simulink model "ACA"  (R2018a)
settings: Solver=FixedStepAuto  StartTime=0.0  StopTime=1000  FixedStep=dt  RelTol=1e-3
InitFcn:
  | ACA_init
values from neighbouring files (symbols this model uses):
  G = [eye(5);-eye(5)]    [dir_alloc_sim.m]
  INDX = IN_MAT(k+3,1:m)'    [DAwrap.m]    (also in LPwrap.m = IN_MAT(end,1:m)'; LPwrap_1.m; TESTac.m = zeros(1,NumU); getUperp.m = IN_MAT(end,:)>0.5)
  LPmethod = 0    [LPwrap.m]    (also in LPwrap_1.m; TESTac.m = 10; test.m = 13)
  NumU = 16    [TESTac.m]    (also in test.m)
  uMax = uMax-ue    [DPnewprio_LPCA.m]    (also in DPscaledprio_LPCA.m; LPwrap.m = umax_act; LPwrap_1.m = umax_act; LPwraparm.m = IN_MAT(5,1:4)')
  uMin = uMin-ue    [DPnewprio_LPCA.m]    (also in DPscaledprio_LPCA.m; LPwrap.m = umin_act; LPwrap_1.m = umin_act; LPwraparm.m = IN_MAT(4,1:4)')
undefined symbols (not defined in the file or in its folder): CAmethod, CB, CGIwrap, d2r, DAwrap, DiscIntNeverNeededParam, dt, LPwrap, M_des, PD_max, PD_min, r2d, u0new, u_max, u_min, UD_max, UD_min, Urlim, UseRL, VD_max, VD_min, VJAwrap, WD_max, WD_min, Wp_aca
libraries: simulink x6
settings Model: Creator=Meng Chaoheng  LastModifiedBy=Meng Chaoheng
settings ModelReferenceCC: ModelReferenceNumInstancesAllowed=Single

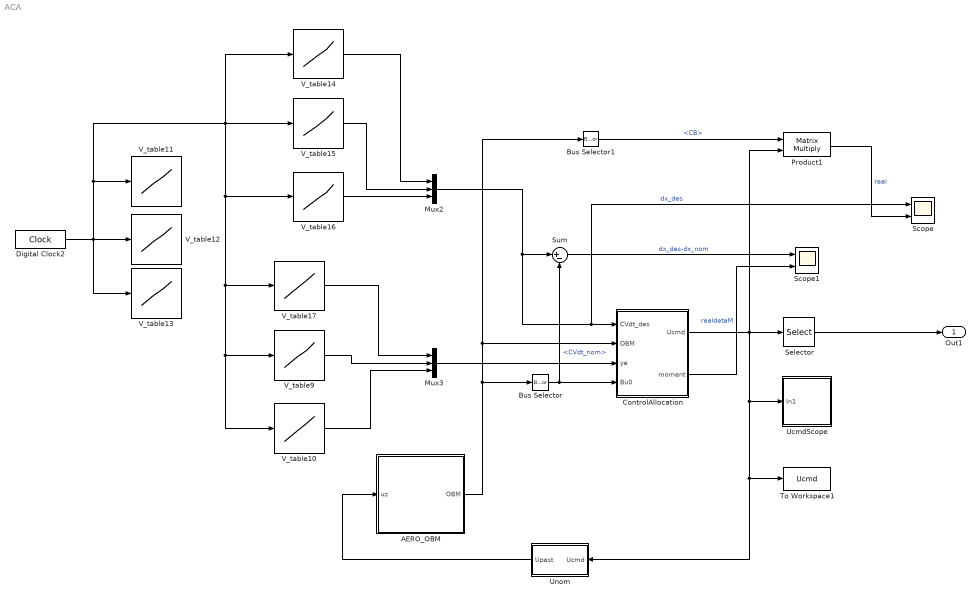
== system ACA ==
  AERO_OBM : Subsystem
  Bus Selector : BusSelector  OutputSignals=CVdt_nom
  Bus Selector1 : BusSelector  OutputSignals=CB
  ControlAllocation : Subsystem
  Digital Clock2 : DigitalClock  SampleTime=dt
  Mux2 : Mux  Inputs=3
  Mux3 : Mux  Inputs=3
  Product1 : Product  Inputs=**  Multiplication=Matrix(*)  RndMeth=Zero
  Scope : Scope  NumInputPorts=2
  Scope1 : Scope  NumInputPorts=2
  Selector : Selector  InputPortWidth=16  IndexOptions=Index vector (dialog)  Indices=[1:4]  OutputSizes=1
  Sum : Sum  Inputs=|+-
  To Workspace1 : ToWorkspace  VariableName=Ucmd  SampleTime=-1
  UcmdScope : Subsystem
  Unom : Subsystem
  V_table10 : Lookup  InputValues=t  Table=ones(length(t),1)*0.0  LookUpMeth=Interpolation-Use End Values
  V_table11 : Lookup  InputValues=t  Table=M_des(:,1)  LookUpMeth=Interpolation-Use End Values
  V_table12 : Lookup  InputValues=t  Table=M_des(:,2)  LookUpMeth=Interpolation-Use End Values
  V_table13 : Lookup  InputValues=t  Table=M_des(:,3)  LookUpMeth=Interpolation-Use End Values
  V_table14 : Lookup  InputValues=t  Table=0.2*sin(0.01*pi*t)  LookUpMeth=Interpolation-Use End Values
  V_table15 : Lookup  InputValues=t  Table=0.2*cos(0.01*pi*t)  LookUpMeth=Interpolation-Use End Values
  V_table16 : Lookup  InputValues=t  Table=0.0*cos(0.02*pi*t)  LookUpMeth=Interpolation-Use End Values
  V_table17 : Lookup  InputValues=t  Table=ones(length(t),1)*0  LookUpMeth=Interpolation-Use End Values
  V_table9 : Lookup  InputValues=t  Table=ones(length(t),1)*0  LookUpMeth=Interpolation-Use End Values
  Out1 : Outport
  wires:
  Unom/1(Upast) -> AERO_OBM/1(uz)
  ControlAllocation/2(moment) -> Scope1/2  "realdetaM"
  Bus Selector/1 -> ControlAllocation/4(Bu0), Sum/2  "<CVdt_nom>"
  AERO_OBM/1(OBM) -> ControlAllocation/2(OBM), Bus Selector1/1, Bus Selector/1
  Bus Selector1/1 -> Product1/1  "<CB>"
  Product1/1 -> Scope/2  "real"
  ControlAllocation/1(Ucmd) -> Product1/2, Selector/1, To Workspace1/1, Unom/1(Ucmd), UcmdScope/1(In1)
  Selector/1 -> Out1/1
  Sum/1 -> Scope1/1  "dx_des-dx_nom"
  Mux3/1 -> ControlAllocation/3(ye)
  Mux2/1 -> ControlAllocation/1(CVdt_des), Scope/1, Sum/1  "dx_des"
  V_table9/1 -> Mux3/2
  V_table17/1 -> Mux3/1
  Digital Clock2/1 -> V_table14/1, V_table15/1, V_table16/1, V_table10/1, V_table9/1, V_table17/1, V_table11/1, V_table13/1, V_table12/1
  V_table14/1 -> Mux2/1
  V_table10/1 -> Mux3/3
  V_table15/1 -> Mux2/2
  V_table16/1 -> Mux2/3

== system ACA/AERO_OBM ==
  uz : Inport
  AeroLimits : Subsystem
  Bus Creator1 : BusCreator  Inputs=5
  Bus Selector : BusSelector  OutputSignals=Unom
  LinearOBM : Subsystem
  OBM : Outport
  wires:
  AeroLimits/1(Umin) -> Bus Creator1/4
  AeroLimits/2(Umax) -> Bus Creator1/5
  Bus Creator1/1 -> OBM/1
  uz/1 -> Bus Selector/1
  Bus Selector/1 -> LinearOBM/1(Unom), Bus Creator1/3  "<Unom>"
  LinearOBM/1(CVdt_nom) -> Bus Creator1/1
  LinearOBM/2(CB) -> Bus Creator1/2

== system ACA/ControlAllocation ==
  CVdt_des : Inport
  OBM : Inport  Port=2
  ye : Inport  Port=3
  Bu0 : Inport  Port=4
  Bus Selector : BusSelector  OutputSignals=CB
  GetU : Subsystem
  PostProcess : Subsystem
  PreProcess : Subsystem
  Product1 : Product  Inputs=**  Multiplication=Matrix(*)  RndMeth=Zero
  Ucmd : Outport
  moment : Outport  Port=2
  wires:
  PreProcess/1(PrePro) -> GetU/1(PrePro), PostProcess/2(PrePro)
  GetU/1(u) -> PostProcess/1(u), Product1/2
  CVdt_des/1 -> PreProcess/1(CVdt_des)  "CVdt_des"
  OBM/1 -> PreProcess/2(OBM), Bus Selector/1
  PostProcess/1(Ucmd) -> Ucmd/1
  Bus Selector/1 -> Product1/1  "<CB>"
  Product1/1 -> moment/1
  ye/1 -> GetU/2(ye)
  Bu0/1 -> GetU/3(Bu0)

== system ACA/UcmdScope ==
  In1 : Inport
  Demux : Demux  Outputs=7
  Selector : Selector  InputPortWidth=16  IndexOptions=Index vector (dialog)  Indices=[1:7]  OutputSizes=1
  Ucmd_deg : Scope  NumInputPorts=7
  scale1 : Gain  Gain=r2d
  wires:
  Selector/1 -> scale1/1
  scale1/1 -> Demux/1
  In1/1 -> Selector/1
  Demux/2 -> Ucmd_deg/2  "LC_deg"
  Demux/1 -> Ucmd_deg/1  "RC_deg"
  Demux/5 -> Ucmd_deg/5  "LIE_deg"
  Demux/7 -> Ucmd_deg/7  "RUD_deg"
  Demux/6 -> Ucmd_deg/6  "LOE_deg"
  Demux/3 -> Ucmd_deg/3  "ROE_deg"
  Demux/4 -> Ucmd_deg/4  "RIE_deg"

== system ACA/Unom ==
  Ucmd : Inport
  Bus Creator : BusCreator  Inputs=2
  Discrete-Time Integrator : DiscreteIntegrator  IntegratorMethod=Integration: Trapezoidal  InitialCondition=u0new  SampleTime=dt  ICPrevOutput=DiscIntNeverNeededParam  ICPrevScaledInput=DiscIntNeverNeededParam
  Get_Unom : Subsystem
  Sum2 : Sum  Inputs=|+-
  Unit Delay1 : UnitDelay  InitialCondition=u0new  SampleTime=dt
  Unit Delay2 : UnitDelay  InitialCondition=u0new  SampleTime=dt
  scale1 : Gain
  scale2 : Gain  Gain=20
  Upast : Outport
  wires:
  Discrete-Time Integrator/1 -> scale1/1, Unit Delay2/1
  Unit Delay1/1 -> Sum2/1, Get_Unom/2(Uz)
  Sum2/1 -> scale2/1
  Unit Delay2/1 -> Sum2/2
  scale2/1 -> Discrete-Time Integrator/1
  Ucmd/1 -> Unit Delay1/1
  scale1/1 -> Get_Unom/1(Uact), Bus Creator/1  "Uact"
  Get_Unom/1(Unom) -> Bus Creator/2
  Bus Creator/1 -> Upast/1

== system ACA/AERO_OBM/AeroLimits ==
  get_uMax : Constant  Value=uMax
  get_uMin : Constant  Value=uMin
  Umin : Outport
  Umax : Outport  Port=2
  wires:
  get_uMin/1 -> Umin/1  "Umin"
  get_uMax/1 -> Umax/1  "Umax"

== system ACA/AERO_OBM/LinearOBM ==
  Unom : Inport
  CB_const : Constant  Value=CB
  Product1 : Product  Inputs=**  Multiplication=Matrix(*)  RndMeth=Zero
  Signal Specification1 : SignalSpecification  Dimensions=[NumU 1]
  CVdt_nom : Outport
  CB : Outport  Port=2
  wires:
  CB_const/1 -> Product1/1, CB/1  "CB"
  Unom/1 -> Signal Specification1/1
  Product1/1 -> CVdt_nom/1  "CVdt_nom"
  Signal Specification1/1 -> Product1/2

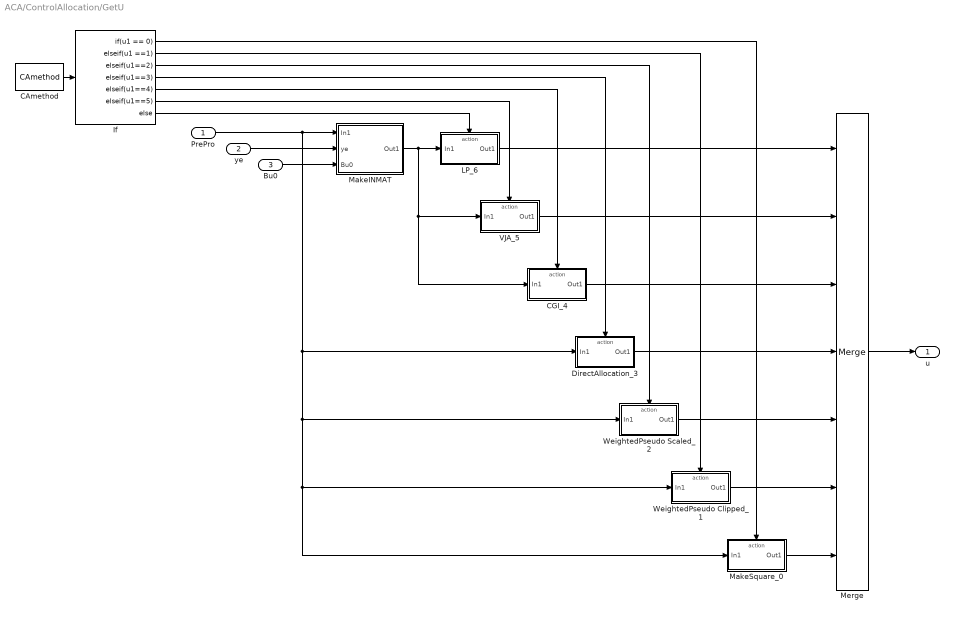
== system ACA/ControlAllocation/GetU ==
  PrePro : Inport
  ye : Inport  Port=2
  Bu0 : Inport  Port=3
  CAmethod : Constant  Value=CAmethod  OutDataTypeStr=int8
  CGI_4 : Subsystem  TreatAsAtomicUnit=on
  DirectAllocation_3 : Subsystem  TreatAsAtomicUnit=on
  If : If  IfExpression=u1 == 0  ElseIfExpressions=u1 ==1, u1==2, u1==3, u1==4, u1==5
  LP_6 : Subsystem  TreatAsAtomicUnit=on
  MakeINMAT : Subsystem
  MakeSquare_0 : Subsystem  TreatAsAtomicUnit=on
  Merge : Merge  Inputs=7
  VJA_5 : Subsystem  TreatAsAtomicUnit=on
  WeightedPseudo Clipped_1 : Subsystem  TreatAsAtomicUnit=on
  WeightedPseudo Scaled_2 : Subsystem  TreatAsAtomicUnit=on
  u : Outport
  wires:
  CAmethod/1 -> If/1
  If/1 -> MakeSquare_0/Action
  If/2 -> WeightedPseudo Clipped_1/Action
  If/3 -> WeightedPseudo Scaled_2/Action
  If/4 -> DirectAllocation_3/Action
  VJA_5/1(Out1) -> Merge/2
  MakeSquare_0/1(Out1) -> Merge/7
  WeightedPseudo Clipped_1/1(Out1) -> Merge/6
  WeightedPseudo Scaled_2/1(Out1) -> Merge/5
  DirectAllocation_3/1(Out1) -> Merge/4
  If/5 -> CGI_4/Action
  CGI_4/1(Out1) -> Merge/3
  If/6 -> VJA_5/Action
  Merge/1 -> u/1
  If/7 -> LP_6/Action
  LP_6/1(Out1) -> Merge/1
  PrePro/1 -> DirectAllocation_3/1(In1), WeightedPseudo Scaled_2/1(In1), WeightedPseudo Clipped_1/1(In1), MakeSquare_0/1(In1), MakeINMAT/1(In1)
  MakeINMAT/1(Out1) -> LP_6/1(In1), VJA_5/1(In1), CGI_4/1(In1)
  ye/1 -> MakeINMAT/2(ye)
  Bu0/1 -> MakeINMAT/3(Bu0)

== system ACA/ControlAllocation/PostProcess ==
  u : Inport
  PrePro : Inport  Port=2
  Bus Selector1 : BusSelector  OutputSignals=Unom
  DriveToPreferred : Subsystem
  Sum2 : Sum  Inputs=|++
  Sum3 : Sum  Inputs=|++
  limits : Subsystem
  Ucmd : Outport
  wires:
  Sum2/1 -> Sum3/1
  u/1 -> DriveToPreferred/2(u), Sum2/1  "u_cmd-u_nom"
  PrePro/1 -> Bus Selector1/1, DriveToPreferred/1(PrePro)
  limits/1(Ucmd) -> Ucmd/1
  Bus Selector1/1 -> Sum2/2  "<Unom>"
  Sum3/1 -> limits/1(In1)
  DriveToPreferred/1(Out2) -> ?

== system ACA/ControlAllocation/PreProcess ==
  CVdt_des : Inport
  OBM : Inport  Port=2
  Bus Creator : BusCreator  Inputs=6
  Bus Selector : BusSelector  OutputSignals=CB
  Bus Selector2 : BusSelector  OutputSignals=Unom
  Constant : Constant  Value=INDX
  GetLimits : Subsystem
  PrePro : Outport
  wires:
  CVdt_des/1 -> Bus Creator/1
  OBM/1 -> Bus Selector/1, Bus Selector2/1, GetLimits/1(OBM)
  Bus Selector/1 -> Bus Creator/2  "<CB>"
  Bus Creator/1 -> PrePro/1
  Bus Selector2/1 -> Bus Creator/3  "<Unom>"
  GetLimits/1(Umin) -> Bus Creator/4
  GetLimits/2(Umax) -> Bus Creator/5
  Constant/1 -> Bus Creator/6  "INDX"

== system ACA/Unom/Get_Unom ==
  note: 2.最优化方法，u_nom是分配起点，
      | 对于典型的QP法，如WLS，SLS等，不要求变量过零，u_nom任意，约束任意，通常无恢复问题（最小范数已经在代价函数中）。
      | 对于LP法，最优化方程的约束只有变量，类似典型QP，约束有方向保持的DP问题：
      | 1）如果u_nom是变化的，即逐帧运行，LP方法有回零恢复问题需要恢复模块（代价函数只优化一帧时）。速度约束可选。
      | 2）如果u_nom是固定点，即全局问题，DP不能加速度约束（不过零）。不需要re可回零，但re可让某些实现的输出曲线更圆滑。
  note: 1.几何法，不考虑约束，和u_nom无关。
  Uact : Inport
  Uz : Inport  Port=2
  Constant3 : Constant  OutDataTypeStr=int8
  Multiport Switch : MultiPortSwitch  Inputs=4
  Utrim : Constant  Value=u0new
  Uzero : Constant  Value=zeros(16,1)
  Unom : Outport
  wires:
  Multiport Switch/1 -> Unom/1  "Unom"
  Constant3/1 -> Multiport Switch/1
  Uzero/1 -> Multiport Switch/2  "Set the nominal values to zero"
  Utrim/1 -> Multiport Switch/3  "Trim the aircraft and use the trimmed values"
  Uz/1 -> Multiport Switch/4  "last computed command"
  Uact/1 -> Multiport Switch/5  "Use the last computed command sent through an estimated effector transfer function"

== system ACA/ControlAllocation/GetU/CGI_4 ==
  In1 : Inport
  Action Port : ActionPort  ActionType=elseif
  MATLAB Fcn : MATLABFcn  MATLABFcn=CGIwrap(u)
  Out1 : Outport
  wires:
  MATLAB Fcn/1 -> Out1/1
  In1/1 -> MATLAB Fcn/1

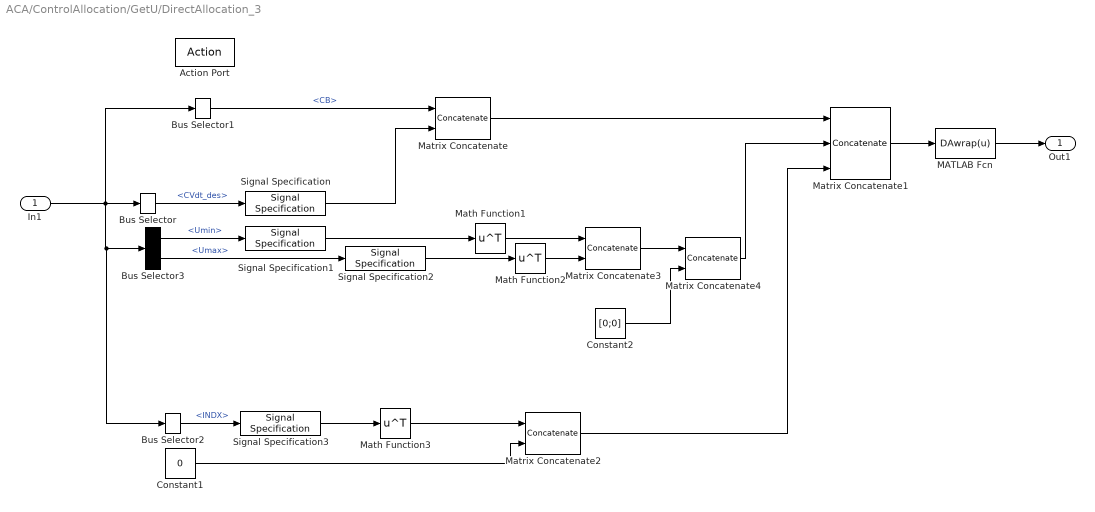
== system ACA/ControlAllocation/GetU/DirectAllocation_3 ==
  In1 : Inport
  Action Port : ActionPort  ActionType=elseif
  Bus Selector : BusSelector  OutputSignals=CVdt_des
  Bus Selector1 : BusSelector  OutputSignals=CB
  Bus Selector2 : BusSelector  OutputSignals=INDX
  Bus Selector3 : BusSelector  OutputSignals=Umin,Umax
  Constant1 : Constant  Value=0
  Constant2 : Constant  Value=[0;0]
  MATLAB Fcn : MATLABFcn  MATLABFcn=DAwrap(u)
  Math Function1 : Math  Operator=transpose  SaturateOnIntegerOverflow=on
  Math Function2 : Math  Operator=transpose  SaturateOnIntegerOverflow=on
  Math Function3 : Math  Operator=transpose  SaturateOnIntegerOverflow=on
  Matrix Concatenate : Concatenate  Mode=Multidimensional array  ConcatenateDimension=2
  Matrix Concatenate1 : Concatenate  NumInputs=3  Mode=Multidimensional array
  Matrix Concatenate2 : Concatenate  Mode=Multidimensional array  ConcatenateDimension=2
  Matrix Concatenate3 : Concatenate  Mode=Multidimensional array
  Matrix Concatenate4 : Concatenate  Mode=Multidimensional array  ConcatenateDimension=2
  Signal Specification : SignalSpecification  Dimensions=[3 1]
  Signal Specification1 : SignalSpecification  Dimensions=[NumU 1]
  Signal Specification2 : SignalSpecification  Dimensions=[NumU 1]
  Signal Specification3 : SignalSpecification  Dimensions=[NumU 1]
  Out1 : Outport
  wires:
  MATLAB Fcn/1 -> Out1/1
  In1/1 -> Bus Selector/1, Bus Selector1/1, Bus Selector2/1, Bus Selector3/1
  Bus Selector/1 -> Signal Specification/1  "<CVdt_des>"
  Bus Selector1/1 -> Matrix Concatenate/1  "<CB>"
  Matrix Concatenate/1 -> Matrix Concatenate1/1
  Matrix Concatenate4/1 -> Matrix Concatenate1/2
  Signal Specification/1 -> Matrix Concatenate/2
  Bus Selector3/1 -> Signal Specification1/1  "<Umin>"
  Bus Selector3/2 -> Signal Specification2/1  "<Umax>"
  Math Function1/1 -> Matrix Concatenate3/1
  Math Function2/1 -> Matrix Concatenate3/2
  Matrix Concatenate3/1 -> Matrix Concatenate4/1
  Constant2/1 -> Matrix Concatenate4/2
  Signal Specification1/1 -> Math Function1/1
  Signal Specification2/1 -> Math Function2/1
  Constant1/1 -> Matrix Concatenate2/2
  Bus Selector2/1 -> Signal Specification3/1  "<INDX>"
  Signal Specification3/1 -> Math Function3/1
  Matrix Concatenate2/1 -> Matrix Concatenate1/3
  Math Function3/1 -> Matrix Concatenate2/1
  Matrix Concatenate1/1 -> MATLAB Fcn/1

== system ACA/ControlAllocation/GetU/LP_6 ==
  In1 : Inport
  Action Port : ActionPort  ActionType=else
  MATLAB Fcn : MATLABFcn  MATLABFcn=LPwrap(u)
  Out1 : Outport
  wires:
  MATLAB Fcn/1 -> Out1/1
  In1/1 -> MATLAB Fcn/1

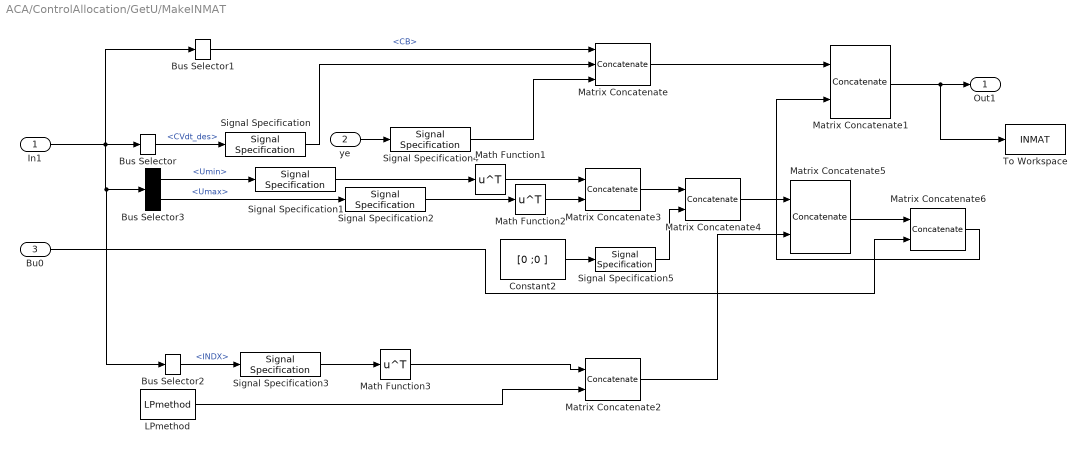
== system ACA/ControlAllocation/GetU/MakeINMAT ==
  In1 : Inport
  ye : Inport  Port=2
  Bu0 : Inport  Port=3
  Bus Selector : BusSelector  OutputSignals=CVdt_des
  Bus Selector1 : BusSelector  OutputSignals=CB
  Bus Selector2 : BusSelector  OutputSignals=INDX
  Bus Selector3 : BusSelector  OutputSignals=Umin,Umax
  Constant2 : Constant  Value=[0 ;0 ]
  LPmethod : Constant  Value=LPmethod
  Math Function1 : Math  Operator=transpose  SaturateOnIntegerOverflow=on
  Math Function2 : Math  Operator=transpose  SaturateOnIntegerOverflow=on
  Math Function3 : Math  Operator=transpose  SaturateOnIntegerOverflow=on
  Matrix Concatenate : Concatenate  NumInputs=3  Mode=Multidimensional array  ConcatenateDimension=2
  Matrix Concatenate1 : Concatenate  Mode=Multidimensional array
  Matrix Concatenate2 : Concatenate  Mode=Multidimensional array  ConcatenateDimension=2
  Matrix Concatenate3 : Concatenate  Mode=Multidimensional array
  Matrix Concatenate4 : Concatenate  Mode=Multidimensional array  ConcatenateDimension=2
  Matrix Concatenate5 : Concatenate  Mode=Multidimensional array
  Matrix Concatenate6 : Concatenate  Mode=Multidimensional array  ConcatenateDimension=2
  Signal Specification : SignalSpecification  Dimensions=[3 1]
  Signal Specification1 : SignalSpecification  Dimensions=[NumU 1]
  Signal Specification2 : SignalSpecification  Dimensions=[NumU 1]
  Signal Specification3 : SignalSpecification  Dimensions=[NumU 1]
  Signal Specification4 : SignalSpecification  Dimensions=[3 1]
  Signal Specification5 : SignalSpecification  Dimensions=[2 1]
  To Workspace : ToWorkspace  VariableName=INMAT  SampleTime=dt
      settings: MaxDataPoints=1
  Out1 : Outport
  wires:
  Math Function3/1 -> Matrix Concatenate2/1
  Matrix Concatenate2/1 -> Matrix Concatenate5/2
  Signal Specification3/1 -> Math Function3/1
  Bus Selector2/1 -> Signal Specification3/1  "<INDX>"
  LPmethod/1 -> Matrix Concatenate2/2
  Signal Specification2/1 -> Math Function2/1
  Signal Specification1/1 -> Math Function1/1
  Constant2/1 -> Signal Specification5/1
  Matrix Concatenate3/1 -> Matrix Concatenate4/1
  Math Function2/1 -> Matrix Concatenate3/2
  Math Function1/1 -> Matrix Concatenate3/1
  Bus Selector3/2 -> Signal Specification2/1  "<Umax>"
  Bus Selector3/1 -> Signal Specification1/1  "<Umin>"
  Signal Specification/1 -> Matrix Concatenate/2
  Matrix Concatenate4/1 -> Matrix Concatenate5/1
  Matrix Concatenate/1 -> Matrix Concatenate1/1
  Bus Selector1/1 -> Matrix Concatenate/1  "<CB>"
  Bus Selector/1 -> Signal Specification/1  "<CVdt_des>"
  In1/1 -> Bus Selector3/1, Bus Selector2/1, Bus Selector1/1, Bus Selector/1
  Matrix Concatenate1/1 -> To Workspace/1, Out1/1
  ye/1 -> Signal Specification4/1
  Signal Specification4/1 -> Matrix Concatenate/3
  Matrix Concatenate5/1 -> Matrix Concatenate6/1
  Bu0/1 -> Matrix Concatenate6/2
  Matrix Concatenate6/1 -> Matrix Concatenate1/2
  Signal Specification5/1 -> Matrix Concatenate4/2

== system ACA/ControlAllocation/GetU/MakeSquare_0 ==
  In1 : Inport
  Action Port : ActionPort  ActionType=then
  Bus Selector2 : BusSelector  OutputSignals=CVdt_des
  Divide : Product  Inputs=*/  Multiplication=Matrix(*)
  Product : Product  Multiplication=Matrix(*)
  Subsystem : Subsystem
  Out1 : Outport
  wires:
  Divide/1 -> Product/1
  Bus Selector2/1 -> Product/2  "<CVdt_des>"
  Product/1 -> Out1/1
  In1/1 -> Bus Selector2/1, Subsystem/1(In1)
  Subsystem/1(Gmod) -> Divide/1
  Subsystem/2(CBGmod) -> Divide/2

== system ACA/ControlAllocation/GetU/VJA_5 ==
  In1 : Inport
  Action Port : ActionPort  ActionType=elseif
  MATLAB Fcn : MATLABFcn  MATLABFcn=VJAwrap(u)
  Out1 : Outport
  wires:
  MATLAB Fcn/1 -> Out1/1
  In1/1 -> MATLAB Fcn/1

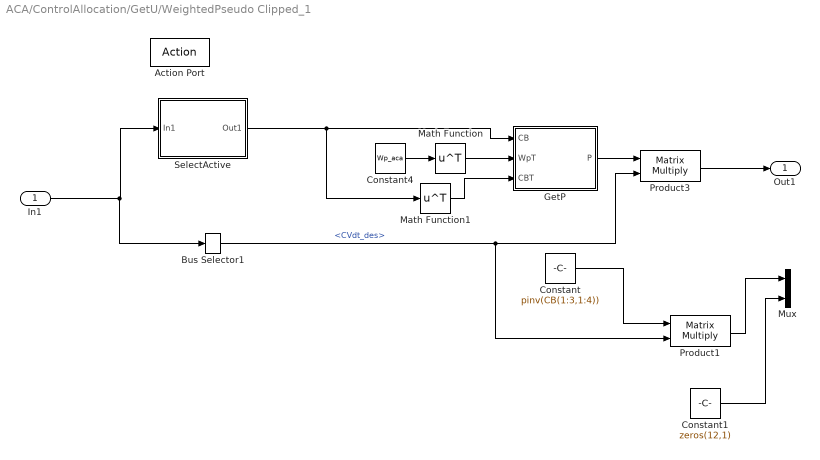
== system ACA/ControlAllocation/GetU/WeightedPseudo Clipped_1 ==
  In1 : Inport
  Action Port : ActionPort  ActionType=elseif
  Bus Selector1 : BusSelector  OutputSignals=CVdt_des
  Constant : Constant  Value=pinv(CB(1:3,1:4))
  Constant1 : Constant  Value=zeros(12,1)
  Constant4 : Constant  Value=Wp_aca
  GetP : Subsystem
  Math Function : Math  Operator=transpose  SaturateOnIntegerOverflow=on
  Math Function1 : Math  Operator=transpose  SaturateOnIntegerOverflow=on
  Mux : Mux  Inputs=2
  Product1 : Product  Inputs=**  Multiplication=Matrix(*)  RndMeth=Zero
  Product3 : Product  Inputs=**  Multiplication=Matrix(*)  RndMeth=Zero
  SelectActive : Subsystem
  Out1 : Outport
  wires:
  Product3/1 -> Out1/1
  Bus Selector1/1 -> Product1/2, Product3/2  "<CVdt_des>"
  GetP/1(P) -> Product3/1
  Math Function1/1 -> GetP/3(CBT)
  Math Function/1 -> GetP/2(WpT)
  Constant4/1 -> Math Function/1
  In1/1 -> Bus Selector1/1, SelectActive/1(In1)
  SelectActive/1(Out1) -> Math Function1/1, GetP/1(CB)
  Constant/1 -> Product1/1
  Product1/1 -> Mux/1
  Constant1/1 -> Mux/2

== system ACA/ControlAllocation/GetU/WeightedPseudo Scaled_2 ==
  In1 : Inport
  Action Port : ActionPort  ActionType=elseif
  Blocks : Subsystem
  Bus Selector1 : BusSelector  OutputSignals=CVdt_des,Umin,Umax
  Constant4 : Constant  Value=Wp_aca
  Gain : Gain
  SelectActive : Subsystem
  Out1 : Outport
  wires:
  Blocks/1(Out1) -> Gain/1
  Constant4/1 -> Blocks/5(Wp)
  Bus Selector1/3 -> Blocks/4(Umax)  "<Umax>"
  Bus Selector1/2 -> Blocks/3(Umin)  "<Umin>"
  Bus Selector1/1 -> Blocks/2(CVdt_des)  "<CVdt_des>"
  Gain/1 -> Out1/1
  In1/1 -> SelectActive/1(In1), Bus Selector1/1
  SelectActive/1(Out1) -> Blocks/1(CB)

== system ACA/ControlAllocation/PostProcess/DriveToPreferred ==
  PrePro : Inport
  u : Inport  Port=2
  Bus Selector2 : BusSelector  OutputSignals=Unom
  Get_UPerp : Subsystem
  LimitScale : Subsystem
  LimitScale1 : Subsystem
  Product : Product  RndMeth=Zero
  Sum2 : Sum
  displaced origin : Subsystem
  Out2 : Outport
  wires:
  u/1 -> displaced origin/1(u), Sum2/2
  PrePro/1 -> Get_UPerp/1(In1), LimitScale1/2(PrePro), LimitScale/4(PrePro), displaced origin/2(PrePro), Bus Selector2/1
  displaced origin/1(MinV) -> LimitScale1/1(MinValues), LimitScale/2(MinValues)
  displaced origin/2(MaxV) -> LimitScale1/3(MaxValues), LimitScale/3(MaxValues)
  Get_UPerp/1(Out1) -> LimitScale1/4(Vector), LimitScale/1(Vector), Product/1  "K_opt * u_perpendicular"
  Product/1 -> Out2/1
  LimitScale1/1(Scale) -> Product/2
  Bus Selector2/1 -> Sum2/1  "<Unom>"
  Sum2/1 -> Get_UPerp/2(In2)

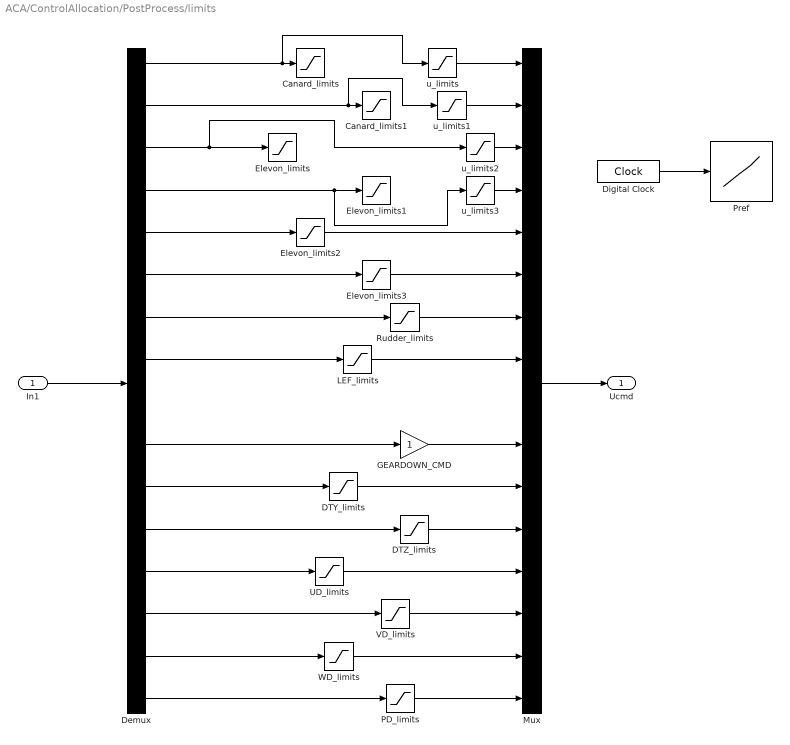
== system ACA/ControlAllocation/PostProcess/limits ==
  In1 : Inport
  Canard_limits : Saturate  UpperLimit=30*d2r  LowerLimit=-30*d2r  RndMeth=Ceiling
  Canard_limits1 : Saturate  UpperLimit=30*d2r  LowerLimit=-30*d2r  RndMeth=Ceiling
  DTY_limits : Saturate  UpperLimit=0.003  LowerLimit=-0.003
  DTZ_limits : Saturate  UpperLimit=0.003  LowerLimit=-0.003
  Demux : Demux  Outputs=16
  Digital Clock : DigitalClock  SampleTime=dt
  Elevon_limits{,1..3} (4 alike) : Saturate  UpperLimit=30*d2r  LowerLimit=-30*d2r  RndMeth=Ceiling
  GEARDOWN_CMD : Gain
  LEF_limits : Saturate  UpperLimit=30*d2r  LowerLimit=-10*d2r  RndMeth=Ceiling
  Mux : Mux  Inputs=16
  PD_limits : Saturate  UpperLimit=PD_max  LowerLimit=PD_min
  Pref : Lookup  InputValues=[0 20 30 40 50 60]  Table=[0 0 0 30 30 30]*d2r  LookUpMeth=Interpolation-Use End Values
  Rudder_limits : Saturate  UpperLimit=30*d2r  LowerLimit=-30*d2r  RndMeth=Ceiling
  UD_limits : Saturate  UpperLimit=UD_max  LowerLimit=UD_min
  VD_limits : Saturate  UpperLimit=VD_max  LowerLimit=VD_min
  WD_limits : Saturate  UpperLimit=WD_max  LowerLimit=WD_min
  u_limits{,1..3} (4 alike) : Saturate  UpperLimit=u_max  LowerLimit=u_min  RndMeth=Ceiling
  Ucmd : Outport
  wires:
  GEARDOWN_CMD/1 -> Mux/10
  Demux/7 -> Rudder_limits/1
  Demux/1 -> u_limits/1, Canard_limits/1
  Elevon_limits2/1 -> Mux/5
  Rudder_limits/1 -> Mux/7
  Demux/6 -> Elevon_limits3/1
  Elevon_limits3/1 -> Mux/6
  Mux/1 -> Ucmd/1
  Demux/3 -> u_limits2/1, Elevon_limits/1
  Demux/2 -> u_limits1/1, Canard_limits1/1
  Demux/5 -> Elevon_limits2/1
  Demux/4 -> u_limits3/1, Elevon_limits1/1
  In1/1 -> Demux/1
  DTY_limits/1 -> Mux/11
  DTZ_limits/1 -> Mux/12
  Demux/11 -> DTY_limits/1
  Demux/12 -> DTZ_limits/1
  Demux/13 -> UD_limits/1
  Demux/14 -> VD_limits/1
  Demux/15 -> WD_limits/1
  Demux/16 -> PD_limits/1
  LEF_limits/1 -> Mux/8
  UD_limits/1 -> Mux/13
  VD_limits/1 -> Mux/14
  WD_limits/1 -> Mux/15
  PD_limits/1 -> Mux/16
  Demux/10 -> GEARDOWN_CMD/1
  Digital Clock/1 -> Pref/1
  Demux/8 -> LEF_limits/1
  u_limits3/1 -> Mux/4
  u_limits2/1 -> Mux/3
  u_limits/1 -> Mux/1
  u_limits1/1 -> Mux/2

== system ACA/ControlAllocation/PreProcess/GetLimits ==
  OBM : Inport
  Constant : Constant  Value=UseRL  OutDataTypeStr=int8
  If : If  IfExpression=u1 == 0
  Merge : Merge
  Merge1 : Merge
  PositionAndRateLimited : Subsystem  TreatAsAtomicUnit=on
  PositionLimited : Subsystem  TreatAsAtomicUnit=on
  Umin : Outport
  Umax : Outport  Port=2
  wires:
  If/1 -> PositionLimited/Action
  If/2 -> PositionAndRateLimited/Action
  PositionAndRateLimited/1(Umin) -> Merge/1
  PositionLimited/2(Umin) -> Merge/2
  PositionAndRateLimited/2(Umax) -> Merge1/1
  PositionLimited/1(Umax) -> Merge1/2
  OBM/1 -> PositionLimited/1(In1), PositionAndRateLimited/1(In1)
  Merge/1 -> Umin/1  "Umin"
  Merge1/1 -> Umax/1  "Umax"
  Constant/1 -> If/1

== system ACA/ControlAllocation/GetU/MakeSquare_0/Subsystem ==
  In1 : Inport
  Bus Selector1 : BusSelector  OutputSignals=CB
  Bus Selector3 : BusSelector  OutputSignals=INDX
  Constant : Constant  Value=G
  Math Function2 : Math  Operator=transpose  SaturateOnIntegerOverflow=on
  Matrix Concatenate : Concatenate  NumInputs=3  Mode=Multidimensional array
  Product : Product
  Product1 : Product  Multiplication=Matrix(*)
  Signal Specification1 : SignalSpecification  Dimensions=[1 NumU]
  Gmod : Outport
  CBGmod : Outport  Port=2
  wires:
  Math Function2/1 -> Product/2
  Bus Selector3/1 -> Signal Specification1/1  "<INDX>"
  Signal Specification1/1 -> Matrix Concatenate/1, Matrix Concatenate/2, Matrix Concatenate/3
  Product/1 -> Product1/2, Gmod/1
  Matrix Concatenate/1 -> Math Function2/1
  Constant/1 -> Product/1
  Bus Selector1/1 -> Product1/1  "<CB>"
  In1/1 -> Bus Selector1/1, Bus Selector3/1
  Product1/1 -> CBGmod/1

== system ACA/ControlAllocation/GetU/WeightedPseudo Clipped_1/GetP ==
  CB : Inport
  WpT : Inport  Port=2
  CBT : Inport  Port=3
  Product : Product  Inputs=/*  Multiplication=Matrix(*)  RndMeth=Zero
  Product1 : Product  Inputs=**  Multiplication=Matrix(*)  RndMeth=Zero
  Product2 : Product  Inputs=*/  Multiplication=Matrix(*)  RndMeth=Zero
  P : Outport
  wires:
  CBT/1 -> Product/2
  Product2/1 -> P/1  "P"
  WpT/1 -> Product/1
  CB/1 -> Product1/1
  Product1/1 -> Product2/2
  Product/1 -> Product2/1, Product1/2

== system ACA/ControlAllocation/GetU/WeightedPseudo Clipped_1/SelectActive ==
  In1 : Inport
  Bus Selector2 : BusSelector  OutputSignals=CB
  Bus Selector3 : BusSelector  OutputSignals=INDX
  Matrix Concatenate : Concatenate  NumInputs=3  Mode=Multidimensional array
  Product : Product
  Signal Specification1 : SignalSpecification  Dimensions=[1 NumU]
  Out1 : Outport
  wires:
  Matrix Concatenate/1 -> Product/1
  Product/1 -> Out1/1
  Bus Selector3/1 -> Signal Specification1/1  "<INDX>"
  Bus Selector2/1 -> Product/2  "<CB>"
  In1/1 -> Bus Selector3/1, Bus Selector2/1
  Signal Specification1/1 -> Matrix Concatenate/3, Matrix Concatenate/2, Matrix Concatenate/1

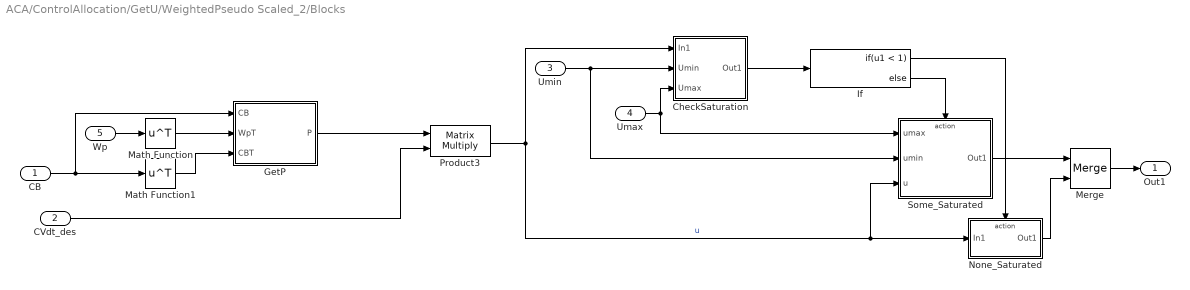
== system ACA/ControlAllocation/GetU/WeightedPseudo Scaled_2/Blocks ==
  CB : Inport
  CVdt_des : Inport  Port=2
  Umin : Inport  Port=3
  Umax : Inport  Port=4
  Wp : Inport  Port=5
  CheckSaturation : Subsystem
  GetP : Subsystem
  If : If  IfExpression=u1 < 1
  Math Function : Math  Operator=transpose  SaturateOnIntegerOverflow=on
  Math Function1 : Math  Operator=transpose  SaturateOnIntegerOverflow=on
  Merge : Merge
  None_Saturated : Subsystem  TreatAsAtomicUnit=on
  Product3 : Product  Inputs=**  Multiplication=Matrix(*)  RndMeth=Zero
  Some_Saturated : Subsystem  TreatAsAtomicUnit=on
  Out1 : Outport
  wires:
  Merge/1 -> Out1/1
  Umin/1 -> Some_Saturated/2(umin), CheckSaturation/2(Umin)
  Umax/1 -> Some_Saturated/1(umax), CheckSaturation/3(Umax)
  None_Saturated/1(Out1) -> Merge/2
  Some_Saturated/1(Out1) -> Merge/1
  If/1 -> None_Saturated/Action
  If/2 -> Some_Saturated/Action
  CheckSaturation/1(Out1) -> If/1
  Product3/1 -> CheckSaturation/1(In1), Some_Saturated/3(u), None_Saturated/1(In1)  "u"
  CVdt_des/1 -> Product3/2
  GetP/1(P) -> Product3/1
  Math Function1/1 -> GetP/3(CBT)
  Math Function/1 -> GetP/2(WpT)
  Wp/1 -> Math Function/1
  CB/1 -> GetP/1(CB), Math Function1/1

== system ACA/ControlAllocation/GetU/WeightedPseudo Scaled_2/SelectActive ==
  In1 : Inport
  Bus Selector2 : BusSelector  OutputSignals=CB
  Bus Selector3 : BusSelector  OutputSignals=INDX
  Matrix Concatenate : Concatenate  NumInputs=3  Mode=Multidimensional array
  Product : Product
  Signal Specification1 : SignalSpecification  Dimensions=[1 NumU]
  Out1 : Outport
  wires:
  Matrix Concatenate/1 -> Product/1
  Product/1 -> Out1/1
  Bus Selector3/1 -> Signal Specification1/1  "<INDX>"
  Bus Selector2/1 -> Product/2  "<CB>"
  In1/1 -> Bus Selector3/1, Bus Selector2/1
  Signal Specification1/1 -> Matrix Concatenate/3, Matrix Concatenate/2, Matrix Concatenate/1

== system ACA/ControlAllocation/PostProcess/DriveToPreferred/Get_UPerp ==
  In1 : Inport
  In2 : Inport  Port=2
  Bus Selector3 : BusSelector  OutputSignals=CB,INDX
  MATLAB Fcn : MATLABFcn  MATLABFcn=getUperp  Output1D=off
  Math Function1 : Math  Operator=transpose  SaturateOnIntegerOverflow=on
  Math Function3 : Math  Operator=transpose  SaturateOnIntegerOverflow=on
  Matrix Concatenate : Concatenate  NumInputs=3  Mode=Multidimensional array
  Signal Specification1 : SignalSpecification  Dimensions=[NumU 1]
  Signal Specification3 : SignalSpecification  Dimensions=[NumU 1]
  Out1 : Outport
  wires:
  Signal Specification3/1 -> Math Function3/1
  Matrix Concatenate/1 -> MATLAB Fcn/1
  In1/1 -> Bus Selector3/1
  Bus Selector3/2 -> Signal Specification3/1  "<INDX>"
  MATLAB Fcn/1 -> Out1/1
  Bus Selector3/1 -> Matrix Concatenate/1  "<CB>"
  In2/1 -> Signal Specification1/1
  Signal Specification1/1 -> Math Function1/1
  Math Function1/1 -> Matrix Concatenate/2
  Math Function3/1 -> Matrix Concatenate/3

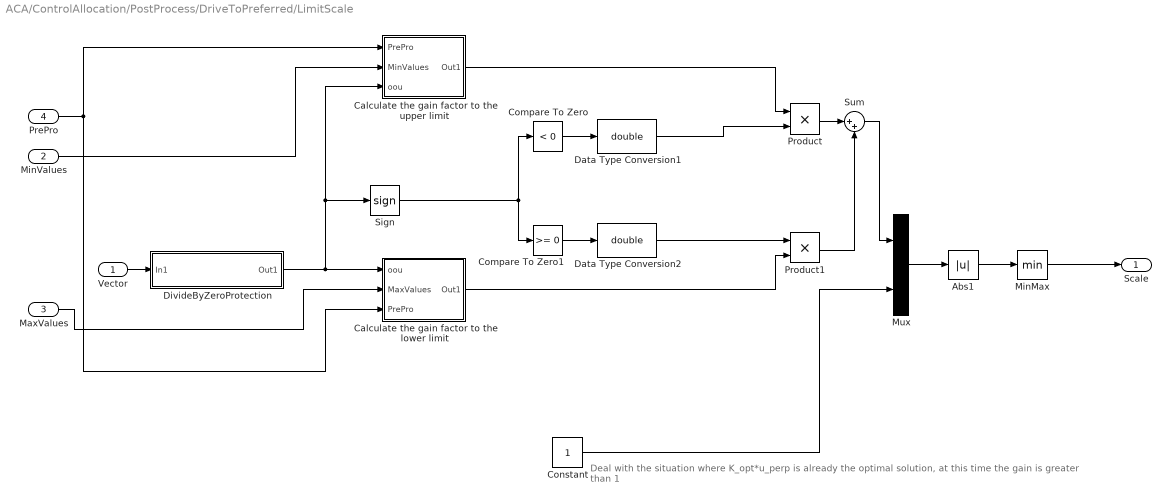
== system ACA/ControlAllocation/PostProcess/DriveToPreferred/LimitScale ==
  note: Deal with the situation where K_opt*u_perp is already the optimal solution, at this time the gain is greater than 1
  Vector : Inport
  MinValues : Inport  Port=2
  MaxValues : Inport  Port=3
  PrePro : Inport  Port=4
  Abs1 : Abs
  "Calculate the gain factor to the lower limit " : Subsystem
  "Calculate the gain factor to the upper limit " : Subsystem
  Compare To Zero : simulink/Logic and Bit Operations/Compare To Zero  relop=<  OutDataTypeStr=uint8
  Compare To Zero1 : simulink/Logic and Bit Operations/Compare To Zero  relop=>=  OutDataTypeStr=uint8
  Constant : Constant
  Data Type Conversion1 : DataTypeConversion  OutDataTypeStr=double
  Data Type Conversion2 : DataTypeConversion  OutDataTypeStr=double
  DivideByZeroProtection : Subsystem
  MinMax : MinMax
  Mux : Mux  Inputs=2
  Product : Product  RndMeth=Zero
  Product1 : Product  RndMeth=Zero
  Sign : Signum
  Sum : Sum  Inputs=|++
  Scale : Outport
  wires:
  Abs1/1 -> MinMax/1
  MinMax/1 -> Scale/1
  Vector/1 -> DivideByZeroProtection/1(In1)
  DivideByZeroProtection/1(Out1) -> "Calculate the gain factor to the lower limit "/1(oou), Sign/1, "Calculate the gain factor to the upper limit "/3(oou)
  Mux/1 -> Abs1/1
  Constant/1 -> Mux/2
  PrePro/1 -> "Calculate the gain factor to the lower limit "/3(PrePro), "Calculate the gain factor to the upper limit "/1(PrePro)
  Sign/1 -> Compare To Zero1/1, Compare To Zero/1
  Compare To Zero/1 -> Data Type Conversion1/1
  Data Type Conversion1/1 -> Product/2
  "Calculate the gain factor to the upper limit "/1(Out1) -> Product/1
  Product/1 -> Sum/1
  Compare To Zero1/1 -> Data Type Conversion2/1
  Data Type Conversion2/1 -> Product1/1
  "Calculate the gain factor to the lower limit "/1(Out1) -> Product1/2
  Product1/1 -> Sum/2
  Sum/1 -> Mux/1
  MaxValues/1 -> "Calculate the gain factor to the lower limit "/2(MaxValues)
  MinValues/1 -> "Calculate the gain factor to the upper limit "/2(MinValues)

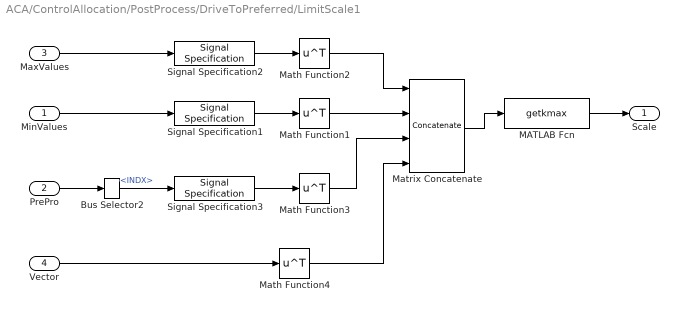
== system ACA/ControlAllocation/PostProcess/DriveToPreferred/LimitScale1 ==
  MinValues : Inport
  PrePro : Inport  Port=2
  MaxValues : Inport  Port=3
  Vector : Inport  Port=4
  Bus Selector2 : BusSelector  OutputSignals=INDX
  MATLAB Fcn : MATLABFcn  MATLABFcn=getkmax  Output1D=off
  Math Function{1..4} (4 alike) : Math  Operator=transpose  SaturateOnIntegerOverflow=on
  Matrix Concatenate : Concatenate  NumInputs=4  Mode=Multidimensional array
  Signal Specification1 : SignalSpecification  Dimensions=[NumU 1]
  Signal Specification2 : SignalSpecification  Dimensions=[NumU 1]
  Signal Specification3 : SignalSpecification  Dimensions=[NumU 1]
  Scale : Outport
  wires:
  PrePro/1 -> Bus Selector2/1
  Vector/1 -> Math Function4/1
  Math Function1/1 -> Matrix Concatenate/2
  Math Function3/1 -> Matrix Concatenate/3
  MinValues/1 -> Signal Specification1/1
  MATLAB Fcn/1 -> Scale/1
  Signal Specification3/1 -> Math Function3/1
  Matrix Concatenate/1 -> MATLAB Fcn/1
  Bus Selector2/1 -> Signal Specification3/1  "<INDX>"
  Signal Specification1/1 -> Math Function1/1
  Signal Specification2/1 -> Math Function2/1
  MaxValues/1 -> Signal Specification2/1
  Math Function2/1 -> Matrix Concatenate/1
  Math Function4/1 -> Matrix Concatenate/4

== system ACA/ControlAllocation/PostProcess/DriveToPreferred/displaced origin ==
  u : Inport
  PrePro : Inport  Port=2
  Bus Selector1 : BusSelector  OutputSignals=Umax
  Bus Selector3 : BusSelector  OutputSignals=Umin
  Sum1 : Sum  Inputs=-+|
  Sum4 : Sum  Inputs=|+-
  MinV : Outport
  MaxV : Outport  Port=2
  wires:
  Bus Selector3/1 -> Sum4/1  "<Umin>"
  PrePro/1 -> Bus Selector3/1, Bus Selector1/1
  Sum4/1 -> MinV/1
  u/1 -> Sum4/2, Sum1/1
  Bus Selector1/1 -> Sum1/2  "<Umax>"
  Sum1/1 -> MaxV/1

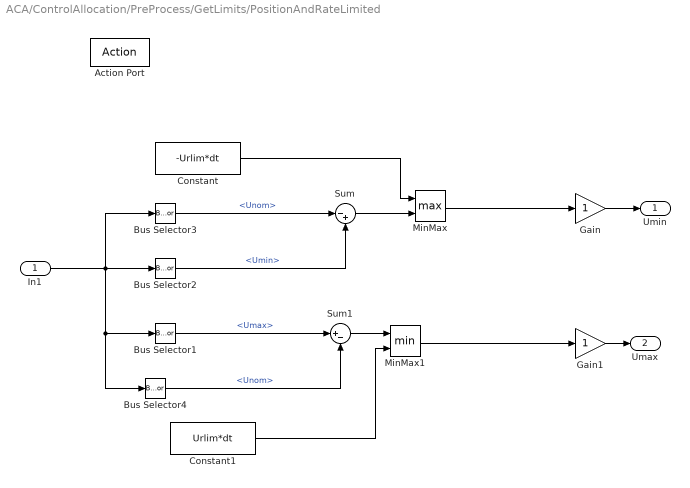
== system ACA/ControlAllocation/PreProcess/GetLimits/PositionAndRateLimited ==
  In1 : Inport
  Action Port : ActionPort  ActionType=else
  Bus Selector1 : BusSelector  OutputSignals=Umax
  Bus Selector2 : BusSelector  OutputSignals=Umin
  Bus Selector3 : BusSelector  OutputSignals=Unom
  Bus Selector4 : BusSelector  OutputSignals=Unom
  Constant : Constant  Value=-Urlim*dt
  Constant1 : Constant  Value=Urlim*dt
  Gain : Gain
  Gain1 : Gain
  MinMax : MinMax  Function=max  Inputs=2
  MinMax1 : MinMax  Inputs=2
  Sum : Sum  Inputs=|-+
  Sum1 : Sum  Inputs=|+-
  Umin : Outport
  Umax : Outport  Port=2
  wires:
  Bus Selector2/1 -> Sum/2  "<Umin>"
  Bus Selector1/1 -> Sum1/1  "<Umax>"
  In1/1 -> Bus Selector2/1, Bus Selector3/1, Bus Selector1/1, Bus Selector4/1
  Gain/1 -> Umin/1
  Gain1/1 -> Umax/1
  Bus Selector3/1 -> Sum/1  "<Unom>"
  Constant/1 -> MinMax/1
  MinMax/1 -> Gain/1
  Sum/1 -> MinMax/2
  Bus Selector4/1 -> Sum1/2  "<Unom>"
  Sum1/1 -> MinMax1/1
  Constant1/1 -> MinMax1/2
  MinMax1/1 -> Gain1/1

== system ACA/ControlAllocation/PreProcess/GetLimits/PositionLimited ==
  In1 : Inport
  Action Port : ActionPort  ActionType=then
  Bus Selector3 : BusSelector  OutputSignals=Umax
  Bus Selector4 : BusSelector  OutputSignals=Umin
  Bus Selector5 : BusSelector  OutputSignals=Unom
  Bus Selector6 : BusSelector  OutputSignals=Unom
  Gain : Gain
  Gain1 : Gain
  Sum : Sum  Inputs=|-+
  Sum1 : Sum  Inputs=|+-
  Umax : Outport
  Umin : Outport  Port=2
  wires:
  Sum/1 -> Gain/1
  Sum1/1 -> Gain1/1
  Gain/1 -> Umin/1
  Gain1/1 -> Umax/1
  Bus Selector4/1 -> Sum/2  "<Umin>"
  Bus Selector3/1 -> Sum1/1  "<Umax>"
  Bus Selector5/1 -> Sum/1  "<Unom>"
  Bus Selector6/1 -> Sum1/2  "<Unom>"
  In1/1 -> Bus Selector5/1, Bus Selector4/1, Bus Selector3/1, Bus Selector6/1

== system ACA/ControlAllocation/GetU/WeightedPseudo Scaled_2/Blocks/CheckSaturation ==
  In1 : Inport
  Umin : Inport  Port=2
  Umax : Inport  Port=3
  Relational Operator : RelationalOperator  Operator=<  OutDataTypeStr=boolean  RndMeth=Nearest
  Relational Operator1 : RelationalOperator  Operator=>  OutDataTypeStr=boolean  RndMeth=Nearest
  Sum : Sum  Inputs=|++
  Sum of Elements : Sum  Inputs=+
  Sum of Elements1 : Sum  Inputs=+
  Out1 : Outport
  wires:
  Sum/1 -> Out1/1
  In1/1 -> Relational Operator/1, Relational Operator1/1
  Sum of Elements1/1 -> Sum/2
  Sum of Elements/1 -> Sum/1
  Relational Operator/1 -> Sum of Elements1/1
  Relational Operator1/1 -> Sum of Elements/1
  Umax/1 -> Relational Operator1/2
  Umin/1 -> Relational Operator/2

== system ACA/ControlAllocation/GetU/WeightedPseudo Scaled_2/Blocks/GetP ==
  CB : Inport
  WpT : Inport  Port=2
  CBT : Inport  Port=3
  Product : Product  Inputs=/*  Multiplication=Matrix(*)  RndMeth=Zero
  Product1 : Product  Inputs=**  Multiplication=Matrix(*)  RndMeth=Zero
  Product2 : Product  Inputs=*/  Multiplication=Matrix(*)  RndMeth=Zero
  P : Outport
  wires:
  CBT/1 -> Product/2
  Product2/1 -> P/1  "P"
  WpT/1 -> Product/1
  CB/1 -> Product1/1
  Product1/1 -> Product2/2
  Product/1 -> Product2/1, Product1/2

== system ACA/ControlAllocation/GetU/WeightedPseudo Scaled_2/Blocks/None_Saturated ==
  In1 : Inport
  Action Port : ActionPort  ActionType=then
  Out1 : Outport
  wires:
  In1/1 -> Out1/1

== system ACA/ControlAllocation/GetU/WeightedPseudo Scaled_2/Blocks/Some_Saturated ==
  umax : Inport
  umin : Inport  Port=2
  u : Inport  Port=3
  Action Port : ActionPort  ActionType=else
  For Iterator Subsystem : Subsystem  TreatAsAtomicUnit=on
  Product : Product  RndMeth=Zero
  Out1 : Outport
  wires:
  Product/1 -> Out1/1
  For Iterator Subsystem/1(Out1) -> Product/2
  umin/1 -> For Iterator Subsystem/3(umin)
  umax/1 -> For Iterator Subsystem/2(umax)
  u/1 -> Product/1, For Iterator Subsystem/1(u)

== system ACA/ControlAllocation/PostProcess/DriveToPreferred/LimitScale/Calculate the gain factor to the lower limit  ==
  oou : Inport
  MaxValues : Inport  Port=2
  PrePro : Inport  Port=3
  Bus Selector2 : BusSelector  OutputSignals=INDX
  Compare To Constant : simulink/Logic and Bit Operations/Compare To Constant  relop=<=  const=0.5  OutDataTypeStr=uint8
  Data Type Conversion : DataTypeConversion  OutDataTypeStr=double
  Product : Product  Inputs=*/  RndMeth=Zero
  Product2 : Product
  Sum : Sum  Inputs=|++
  Out1 : Outport
  wires:
  Compare To Constant/1 -> Data Type Conversion/1
  Data Type Conversion/1 -> Sum/1
  Bus Selector2/1 -> Product2/1, Compare To Constant/1  "<INDX>"
  Product2/1 -> Sum/2
  PrePro/1 -> Bus Selector2/1
  MaxValues/1 -> Product/1
  Sum/1 -> Out1/1
  oou/1 -> Product/2
  Product/1 -> Product2/2  "gain,  K"

== system ACA/ControlAllocation/PostProcess/DriveToPreferred/LimitScale/Calculate the gain factor to the upper limit  ==
  PrePro : Inport
  MinValues : Inport  Port=2
  oou : Inport  Port=3
  Bus Selector2 : BusSelector  OutputSignals=INDX
  Compare To Constant : simulink/Logic and Bit Operations/Compare To Constant  relop=<=  const=0.5  OutDataTypeStr=uint8
  Data Type Conversion : DataTypeConversion  OutDataTypeStr=double
  Product : Product  Inputs=*/  RndMeth=Zero
  Product2 : Product
  Sum : Sum  Inputs=|++
  Out1 : Outport
  wires:
  Product/1 -> Product2/2
  oou/1 -> Product/2
  Sum/1 -> Out1/1
  MinValues/1 -> Product/1
  PrePro/1 -> Bus Selector2/1
  Product2/1 -> Sum/2
  Bus Selector2/1 -> Product2/1, Compare To Constant/1  "<INDX>"
  Data Type Conversion/1 -> Sum/1
  Compare To Constant/1 -> Data Type Conversion/1

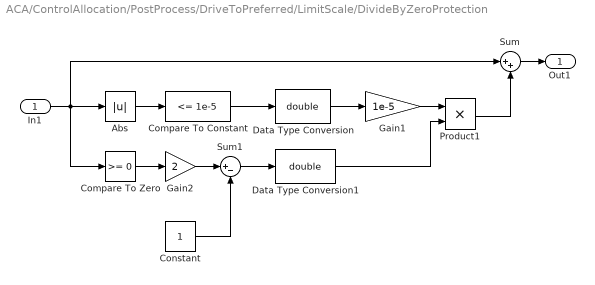
== system ACA/ControlAllocation/PostProcess/DriveToPreferred/LimitScale/DivideByZeroProtection ==
  In1 : Inport
  Abs : Abs
  Compare To Constant : simulink/Logic and Bit Operations/Compare To Constant  relop=<=  const=1e-5  OutDataTypeStr=uint8
  Compare To Zero : simulink/Logic and Bit Operations/Compare To Zero  relop=>=  OutDataTypeStr=uint8
  Constant : Constant
  Data Type Conversion : DataTypeConversion  OutDataTypeStr=double
  Data Type Conversion1 : DataTypeConversion  OutDataTypeStr=double
  Gain1 : Gain  Gain=1e-5
  Gain2 : Gain  Gain=2
  Product1 : Product  RndMeth=Zero
  Sum : Sum  Inputs=|++
  Sum1 : Sum  Inputs=|+-
  Out1 : Outport
  wires:
  Abs/1 -> Compare To Constant/1
  Data Type Conversion/1 -> Gain1/1
  Gain1/1 -> Product1/1
  Sum1/1 -> Data Type Conversion1/1
  Compare To Zero/1 -> Gain2/1
  Gain2/1 -> Sum1/1
  Constant/1 -> Sum1/2
  Data Type Conversion1/1 -> Product1/2
  Compare To Constant/1 -> Data Type Conversion/1
  In1/1 -> Sum/1, Compare To Zero/1, Abs/1
  Product1/1 -> Sum/2
  Sum/1 -> Out1/1

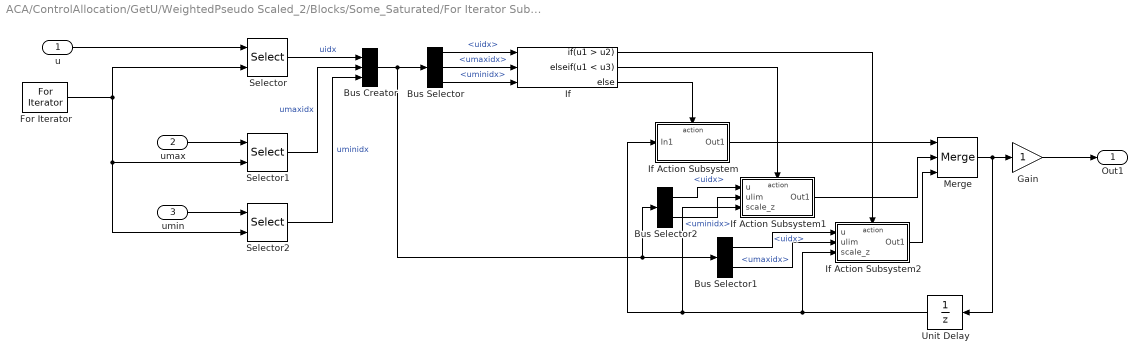
== system ACA/ControlAllocation/GetU/WeightedPseudo Scaled_2/Blocks/Some_Saturated/For Iterator Subsystem ==
  u : Inport
  umax : Inport  Port=2
  umin : Inport  Port=3
  Bus Creator : BusCreator  Inputs=3
  Bus Selector : BusSelector  OutputSignals=uidx,umaxidx,uminidx
  Bus Selector1 : BusSelector  OutputSignals=uidx,umaxidx
  Bus Selector2 : BusSelector  OutputSignals=uidx,uminidx
  For Iterator : ForIterator  IterationLimit=7
  Gain : Gain
  If : If  NumInputs=3  IfExpression=u1 > u2  ElseIfExpressions=u1 < u3
  If Action Subsystem : Subsystem  TreatAsAtomicUnit=on
  If Action Subsystem1 : Subsystem  TreatAsAtomicUnit=on
  If Action Subsystem2 : Subsystem  TreatAsAtomicUnit=on
  Merge : Merge  Inputs=3
  Selector : Selector  IndexOptions=Index vector (port)  Indices=[1 3]  OutputSizes=1
  Selector1 : Selector  IndexOptions=Index vector (port)  Indices=[1 3]  OutputSizes=1
  Selector2 : Selector  IndexOptions=Index vector (port)  Indices=[1 3]  OutputSizes=1
  Unit Delay : UnitDelay  InitialCondition=1  SampleTime=-1
  Out1 : Outport
  wires:
  Bus Selector2/2 -> If Action Subsystem1/2(ulim)  "<uminidx>"
  Bus Selector2/1 -> If Action Subsystem1/1(u)  "<uidx>"
  Bus Selector1/2 -> If Action Subsystem2/2(ulim)  "<umaxidx>"
  Bus Selector1/1 -> If Action Subsystem2/1(u)  "<uidx>"
  Bus Selector/3 -> If/3  "<uminidx>"
  Bus Selector/2 -> If/2  "<umaxidx>"
  Bus Selector/1 -> If/1  "<uidx>"
  Bus Creator/1 -> Bus Selector2/1, Bus Selector1/1, Bus Selector/1
  Unit Delay/1 -> If Action Subsystem1/3(scale_z), If Action Subsystem/1(In1), If Action Subsystem2/3(scale_z)
  Merge/1 -> Unit Delay/1, Gain/1
  If Action Subsystem1/1(Out1) -> Merge/2
  If Action Subsystem2/1(Out1) -> Merge/3
  If Action Subsystem/1(Out1) -> Merge/1
  If/1 -> If Action Subsystem2/Action
  If/2 -> If Action Subsystem1/Action
  If/3 -> If Action Subsystem/Action
  Selector2/1 -> Bus Creator/3  "uminidx"
  Selector1/1 -> Bus Creator/2  "umaxidx"
  Selector/1 -> Bus Creator/1  "uidx"
  umin/1 -> Selector2/1
  umax/1 -> Selector1/1
  Gain/1 -> Out1/1
  For Iterator/1 -> Selector2/2, Selector1/2, Selector/2
  u/1 -> Selector/1

== system ACA/ControlAllocation/GetU/WeightedPseudo Scaled_2/Blocks/Some_Saturated/For Iterator Subsystem/If Action Subsystem ==
  In1 : Inport
  Action Port : ActionPort  ActionType=else
  Out1 : Outport
  wires:
  In1/1 -> Out1/1

== system ACA/ControlAllocation/GetU/WeightedPseudo Scaled_2/Blocks/Some_Saturated/For Iterator Subsystem/If Action Subsystem1 ==
  u : Inport
  ulim : Inport  Port=2
  scale_z : Inport  Port=3
  Action Port : ActionPort  ActionType=elseif
  Abs : Abs
  If : If  IfExpression=u1 >1e-5
  If Action Subsystem : Subsystem  TreatAsAtomicUnit=on
  If Action Subsystem1 : Subsystem  TreatAsAtomicUnit=on
  Merge : Merge
  Out1 : Outport
  wires:
  If Action Subsystem/1(Out1) -> Merge/2
  If/1 -> If Action Subsystem/Action
  If Action Subsystem1/1(Out1) -> Merge/1
  If/2 -> If Action Subsystem1/Action
  scale_z/1 -> If Action Subsystem/3(scale_z)
  ulim/1 -> If Action Subsystem/2(ulim)
  Merge/1 -> Out1/1
  u/1 -> If Action Subsystem/1(u), Abs/1
  Abs/1 -> If/1

== system ACA/ControlAllocation/GetU/WeightedPseudo Scaled_2/Blocks/Some_Saturated/For Iterator Subsystem/If Action Subsystem2 ==
  u : Inport
  ulim : Inport  Port=2
  scale_z : Inport  Port=3
  Action Port : ActionPort  ActionType=then
  Abs : Abs
  If : If  IfExpression=u1 >1e-5
  If Action Subsystem : Subsystem  TreatAsAtomicUnit=on
  If Action Subsystem1 : Subsystem  TreatAsAtomicUnit=on
  Merge : Merge
  Out1 : Outport
  wires:
  If Action Subsystem/1(Out1) -> Merge/2
  If/1 -> If Action Subsystem/Action
  If Action Subsystem1/1(Out1) -> Merge/1
  If/2 -> If Action Subsystem1/Action
  scale_z/1 -> If Action Subsystem/3(scale_z)
  ulim/1 -> If Action Subsystem/2(ulim)
  Merge/1 -> Out1/1
  u/1 -> If Action Subsystem/1(u), Abs/1
  Abs/1 -> If/1

== system ACA/ControlAllocation/GetU/WeightedPseudo Scaled_2/Blocks/Some_Saturated/For Iterator Subsystem/If Action Subsystem1/If Action Subsystem ==
  u : Inport
  ulim : Inport  Port=2
  scale_z : Inport  Port=3
  Action Port : ActionPort  ActionType=then
  MinMax : MinMax  Inputs=2
  Product : Product  Inputs=*/  RndMeth=Zero
  Out1 : Outport
  wires:
  MinMax/1 -> Out1/1
  Product/1 -> MinMax/1
  u/1 -> Product/2
  ulim/1 -> Product/1
  scale_z/1 -> MinMax/2

== system ACA/ControlAllocation/GetU/WeightedPseudo Scaled_2/Blocks/Some_Saturated/For Iterator Subsystem/If Action Subsystem1/If Action Subsystem1 ==
  Action Port : ActionPort  ActionType=else
  Constant4 : Constant  Value=0
  Out1 : Outport
  wires:
  Constant4/1 -> Out1/1

== system ACA/ControlAllocation/GetU/WeightedPseudo Scaled_2/Blocks/Some_Saturated/For Iterator Subsystem/If Action Subsystem2/If Action Subsystem ==
  u : Inport
  ulim : Inport  Port=2
  scale_z : Inport  Port=3
  Action Port : ActionPort  ActionType=then
  MinMax : MinMax  Inputs=2
  Product : Product  Inputs=*/  RndMeth=Zero
  Out1 : Outport
  wires:
  MinMax/1 -> Out1/1
  Product/1 -> MinMax/1
  u/1 -> Product/2
  ulim/1 -> Product/1
  scale_z/1 -> MinMax/2

== system ACA/ControlAllocation/GetU/WeightedPseudo Scaled_2/Blocks/Some_Saturated/For Iterator Subsystem/If Action Subsystem2/If Action Subsystem1 ==
  Action Port : ActionPort  ActionType=else
  Constant4 : Constant  Value=0
  Out1 : Outport
  wires:
  Constant4/1 -> Out1/1
